simulink model "CLRFSPFCRealizedSimscape"  (R2024a)
settings: Solver=FixedStepAuto  StartTime=0.0  StopTime=0.1  FixedStep=1e-7  MaxStep=1e-6  RelTol=1e-3
undefined symbols (not defined in the file or in its folder): Rc1, Rc2, Rc3, Rclp, Rin1, Rin2, Rin3, Rout, Rst1, Rst2, Vc, vr
libraries: fl_lib x44, nesl_utility x9, ee_lib x5
settings Model: Creator=FactCore  LastModifiedBy=FactCore
settings SolverCC: ZeroCrossAlgorithm=Adaptive

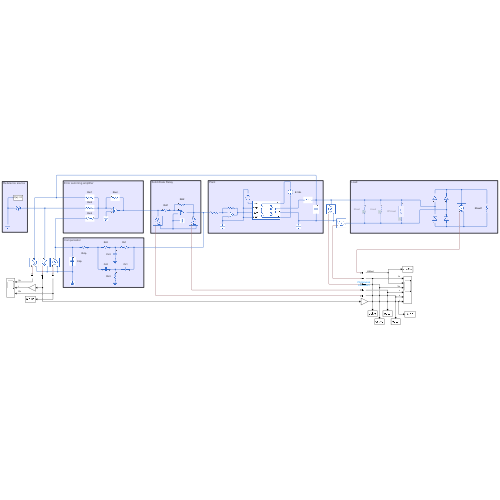
[thumbnail: Simulink's stored preview of the top-level diagram]
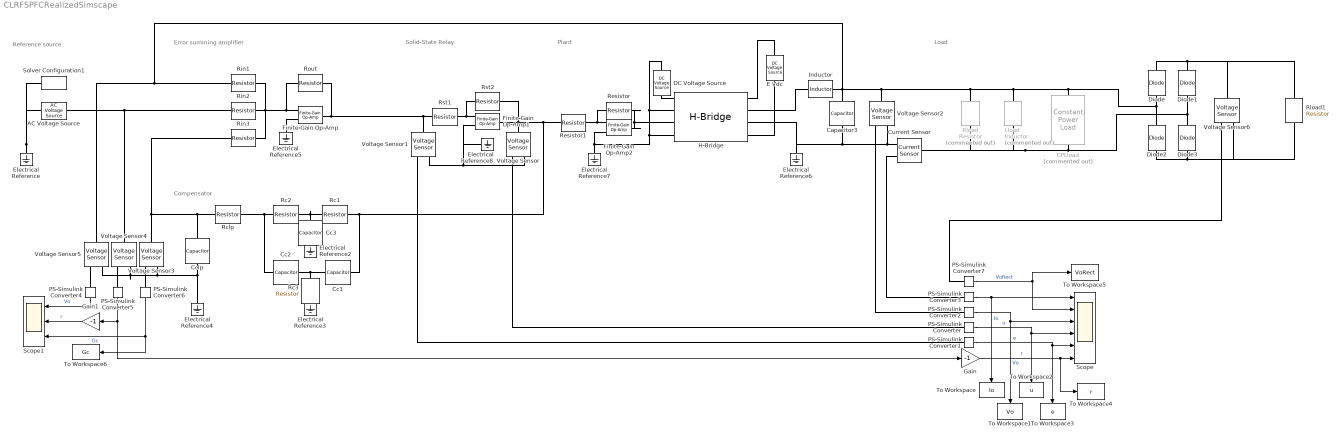
== system CLRFSPFCRealizedSimscape ==
  note: Reference source
  note: Error summing amplifier
  note: Compensator
  note: Load
  note: Plant
  note: Solid-State Relay
  AC Voltage Source : fl_lib/Electrical/Electrical Sources/AC Voltage Source  amp=vr*sqrt(2) V  shift=0 deg  frequency=fg Hz
  CPLload : ee_lib/Passive/Constant Power Load  Commented=on  load_type=ee.enum.dc_ac.ac  consumed_power=100 W  min_supply_voltage=20 V  G_reverse=1e-6 S  deltaV=1e-3 V  active_power=400 W  reactive_power=0 A*V  f0=fg Hz  Vrms_min=vr*0.85 V  tau=0.01 s  Vrms_ini=vr V  Vang_ini=0 deg  enable_fault=simscape.enum.onoff.off  fault_action=simscape.enum.assert.action.none  t_fault=1 s  open_conductance=1e-4 S
      settings: InternalSimscapePortConfiguration="{\"Bottom\":[],\"Left\":[{\"id\":\"p\",\"label\":\"+\",\"type\":\"foundation.electrical.electrical\"}],\"Right\":[{\"id\":\"n\",\"label\":\"-\",\"type\":\"foundation.electrical.electrical\"}],\"Top\":[]}"
  Capacitor3 : fl_lib/Electrical/Electrical Elements/Capacitor  c=Cf F  r=1e-6 Ohm  g=0 1/Ohm  i_specify=off  i_priority=None  i=0 A  i_nominal_specify=off  i_nominal_value=1  i_nominal_unit=A  v_specify=off  v_priority=None  v=0 V  v_nominal_specify=off  v_nominal_value=1  v_nominal_unit=V  vc_specify=off  vc_priority=High  vc=0 V  vc_nominal_specify=off  vc_nominal_value=1  vc_nominal_unit=V
  Cc1 : fl_lib/Electrical/Electrical Elements/Capacitor  c=Cc1 F  r=1e-6 Ohm  g=0 1/Ohm  i_specify=off  i_priority=None  i=0 A  i_nominal_specify=off  i_nominal_value=1  i_nominal_unit=A  v_specify=off  v_priority=None  v=0 V  v_nominal_specify=off  v_nominal_value=1  v_nominal_unit=V  vc_specify=off  vc_priority=High  vc=0 V  vc_nominal_specify=off  vc_nominal_value=1  vc_nominal_unit=V
  Cc2 : fl_lib/Electrical/Electrical Elements/Capacitor  c=Cc2 F  r=1e-6 Ohm  g=0 1/Ohm  i_specify=off  i_priority=None  i=0 A  i_nominal_specify=off  i_nominal_value=1  i_nominal_unit=A  v_specify=off  v_priority=None  v=0 V  v_nominal_specify=off  v_nominal_value=1  v_nominal_unit=V  vc_specify=off  vc_priority=High  vc=0 V  vc_nominal_specify=off  vc_nominal_value=1  vc_nominal_unit=V
  Cc3 : fl_lib/Electrical/Electrical Elements/Capacitor  c=Cc3 F  r=1e-6 Ohm  g=0 1/Ohm  i_specify=off  i_priority=None  i=0 A  i_nominal_specify=off  i_nominal_value=1  i_nominal_unit=A  v_specify=off  v_priority=None  v=0 V  v_nominal_specify=off  v_nominal_value=1  v_nominal_unit=V  vc_specify=off  vc_priority=High  vc=0 V  vc_nominal_specify=off  vc_nominal_value=1  vc_nominal_unit=V
  Cclp : fl_lib/Electrical/Electrical Elements/Capacitor  c=Cclp F  r=1e-6 Ohm  g=0 1/Ohm  i_specify=off  i_priority=None  i=0 A  i_nominal_specify=off  i_nominal_value=1  i_nominal_unit=A  v_specify=off  v_priority=None  v=0 V  v_nominal_specify=off  v_nominal_value=1  v_nominal_unit=V  vc_specify=off  vc_priority=High  vc=0 V  vc_nominal_specify=off  vc_nominal_value=1  vc_nominal_unit=V
  Current Sensor : fl_lib/Electrical/Electrical Sensors/Current Sensor
  DC Voltage Source : fl_lib/Electrical/Electrical Sources/DC Voltage Source  v0=5 V
  Diode{,1..3} (4 alike) : fl_lib/Electrical/Electrical Elements/Diode  Vf=0.6 V  Ron=0.3 Ohm  Goff=1e-8 1/Ohm  i_specify=off  i_priority=None  i=0 A  i_nominal_specify=off  i_nominal_value=1  i_nominal_unit=A  v_specify=off  v_priority=None  v=0 V  v_nominal_specify=off  v_nominal_value=1  v_nominal_unit=V
  E Vdc : fl_lib/Electrical/Electrical Sources/DC Voltage Source  v0=E V
  Electrical Reference{,2..8} (8 alike) : fl_lib/Electrical/Electrical Elements/Electrical Reference
  Finite-Gain Op-Amp : ee_lib/Integrated Circuits/Finite-Gain Op-Amp  A=1e4  Rin=1e6 Ohm  Rout=0.3 Ohm  Vmin=-Vc V  Vmax=Vc V  noise_mode=ee.enum.mode.disabled  v_noise=30e-9 V/Hz^(1/2)  noise_prm=ee.enum.ic.noiseParameterization.same  i_noise=0.5e-12 A/Hz^(1/2)  ip_noise=0.5e-12 A/Hz^(1/2)  in_noise=0.5e-12 A/Hz^(1/2)  sample_time=1e-3 s  repeatability=ee.enum.ic.repeatability.notRepeatable  auto_seed_v=545404223  auto_seed_ip=3922919431  auto_seed_in=2715962282  user_seed_v=0  user_seed_ip=0  user_seed_in=0
      settings: InternalSimscapePortConfiguration="{\"Bottom\":[],\"Left\":[{\"id\":\"p\",\"label\":\"+\",\"type\":\"foundation.electrical.electrical\"},{\"id\":\"n\",\"label\":\"-\",\"type\":\"foundation.electrical.electrical\"}],\"Right\":[{\"id\":\"out\",\"label\":\"\",\"type\":\"foundation.electrical.electrical\"}],\"Top\":[]}"
  Finite-Gain Op-Amp1 : ee_lib/Integrated Circuits/Finite-Gain Op-Amp  A=1e9  Rin=1e6 Ohm  Rout=0.3 Ohm  Vmin=-Vc V  Vmax=Vc V  noise_mode=ee.enum.mode.disabled  v_noise=30e-9 V/Hz^(1/2)  noise_prm=ee.enum.ic.noiseParameterization.same  i_noise=0.5e-12 A/Hz^(1/2)  ip_noise=0.5e-12 A/Hz^(1/2)  in_noise=0.5e-12 A/Hz^(1/2)  sample_time=1e-3 s  repeatability=ee.enum.ic.repeatability.notRepeatable  auto_seed_v=3437178441  auto_seed_ip=609397185  auto_seed_in=1811450916  user_seed_v=0  user_seed_ip=0  user_seed_in=0
      settings: InternalSimscapePortConfiguration="{\"Bottom\":[],\"Left\":[{\"id\":\"p\",\"label\":\"+\",\"type\":\"foundation.electrical.electrical\"},{\"id\":\"n\",\"label\":\"-\",\"type\":\"foundation.electrical.electrical\"}],\"Right\":[{\"id\":\"out\",\"label\":\"\",\"type\":\"foundation.electrical.electrical\"}],\"Top\":[]}"
  Finite-Gain Op-Amp2 : ee_lib/Integrated Circuits/Finite-Gain Op-Amp  A=1e4  Rin=1e6 Ohm  Rout=0.3 Ohm  Vmin=-Vc V  Vmax=Vc V  noise_mode=ee.enum.mode.disabled  v_noise=30e-9 V/Hz^(1/2)  noise_prm=ee.enum.ic.noiseParameterization.same  i_noise=0.5e-12 A/Hz^(1/2)  ip_noise=0.5e-12 A/Hz^(1/2)  in_noise=0.5e-12 A/Hz^(1/2)  sample_time=1e-3 s  repeatability=ee.enum.ic.repeatability.notRepeatable  auto_seed_v=2348838240  auto_seed_ip=4112460543  auto_seed_in=4144164703  user_seed_v=0  user_seed_ip=0  user_seed_in=0
      settings: InternalSimscapePortConfiguration="{\"Bottom\":[],\"Left\":[{\"id\":\"p\",\"label\":\"+\",\"type\":\"foundation.electrical.electrical\"},{\"id\":\"n\",\"label\":\"-\",\"type\":\"foundation.electrical.electrical\"}],\"Right\":[{\"id\":\"out\",\"label\":\"\",\"type\":\"foundation.electrical.electrical\"}],\"Top\":[]}"
  Gain : Gain  Gain=-1
  Gain1 : Gain  Gain=-1
  H-Bridge : ee_lib/Semiconductors & Converters/Converters/H-Bridge  supply_ports=ee.enum.supply_ports.showsupply  pwm_or_av=ee.enum.pwm_or_av.pwm  regenerative_braking_mode=ee.enum.converters.regenerative_braking_mode.depends_on_rev  discontinuous=ee.enum.current_profile.continuous  freewheeling_mode=ee.enum.converters.freewheeling_mode.one_switch_one_diode  Rload=10 Ohm  Lload=1e-5 H  F=10 kHz  Venable=2.5 V  Vmax=5.0 V  Vreverse=0.1 V  Vbrake=2.5 V  Vm=12 V  Ron=0.1 Ohm  Don=0.05 Ohm  Goff=1e-6 S  Tmeas=298.15 K  Ron2=0.1 Ohm  Don2=0.05 Ohm  Tmeas2=398.15 K  thermal_mass=100 J/K  initial_temperature=298.15 K
      settings: InternalSimscapePortConfiguration="{\"Bottom\":[],\"Left\":[{\"id\":\"ENA\",\"label\":\"PWM\",\"type\":\"foundation.electrical.electrical\"},{\"id\":\"REF\",\"label\":\"REF\",\"type\":\"foundation.electrical.electrical\"},{\"id\":\"REV\",\"label\":\"REV\",\"type\":\"foundation.electrical.electrical\"},{\"id\":\"BRK\",\"label\":\"BRK\",\"type\":\"foundation.electrical.electrical\"}],\"Right\":[{\"id\":\"p1\",\"label\":\"V+\",\"type\":\"foundation.electrical.electrical\"},{\"id\":\"p2\",\"label\":\"+\",\"type\":\"foundation.electrical.electrical\"},{\"id\":\"n2\",\"label\":\"-\",\"type\":\"foundation.electrical.electrical\"},{\"id\":\"n1\",\"label\":\"V-\",\"type\":\"foundation.electrical.electrical\"}],\"Top\":[]}"
  Inductor : fl_lib/Electrical/Electrical Elements/Inductor  l=Lf H  r=Rf Ohm  g=1e-9 1/Ohm  i_specify=off  i_priority=None  i=0 A  i_nominal_specify=off  i_nominal_value=1  i_nominal_unit=A  v_specify=off  v_priority=None  v=0 V  v_nominal_specify=off  v_nominal_value=1  v_nominal_unit=V  i_L_specify=off  i_L_priority=High  i_L=0 A  i_L_nominal_specify=off  i_L_nominal_value=1  i_L_nominal_unit=A
  Lload : fl_lib/Electrical/Electrical Elements/Inductor  Commented=on  l=400e-3 H  r=1 Ohm  g=1e-9 1/Ohm  i_specify=off  i_priority=None  i=0 A  i_nominal_specify=off  i_nominal_value=1  i_nominal_unit=A  v_specify=off  v_priority=None  v=0 V  v_nominal_specify=off  v_nominal_value=1  v_nominal_unit=V  i_L_specify=off  i_L_priority=High  i_L=0 A  i_L_nominal_specify=off  i_L_nominal_value=1  i_L_nominal_unit=A
  PS-Simulink Converter{,1..7} (8 alike) : nesl_utility/PS-Simulink Converter  PhysicalDomain=network_engine_domain  SubClassName=ps_output  LeftPortType=input  RightPortType=output  PseudoPeriodic=off  Frequencies=[]  VectorFormat=inherit  Unit=inherit  AffineConversion=off
  Rc1 : fl_lib/Electrical/Electrical Elements/Resistor  R=Rc1 Ohm  i_specify=off  i_priority=None  i=0 A  i_nominal_specify=off  i_nominal_value=1  i_nominal_unit=A  v_specify=off  v_priority=None  v=0 V  v_nominal_specify=off  v_nominal_value=1  v_nominal_unit=V
  Rc2 : fl_lib/Electrical/Electrical Elements/Resistor  R=Rc2 Ohm  i_specify=off  i_priority=None  i=0 A  i_nominal_specify=off  i_nominal_value=1  i_nominal_unit=A  v_specify=off  v_priority=None  v=0 V  v_nominal_specify=off  v_nominal_value=1  v_nominal_unit=V
  Rc3 : fl_lib/Electrical/Electrical Elements/Resistor  R=Rc3 Ohm  i_specify=off  i_priority=None  i=0 A  i_nominal_specify=off  i_nominal_value=1  i_nominal_unit=A  v_specify=off  v_priority=None  v=0 V  v_nominal_specify=off  v_nominal_value=1  v_nominal_unit=V
  Rclp : fl_lib/Electrical/Electrical Elements/Resistor  R=Rclp Ohm  i_specify=off  i_priority=None  i=0 A  i_nominal_specify=off  i_nominal_value=1  i_nominal_unit=A  v_specify=off  v_priority=None  v=0 V  v_nominal_specify=off  v_nominal_value=1  v_nominal_unit=V
  Resistor : fl_lib/Electrical/Electrical Elements/Resistor  R=10e3 Ohm  i_specify=off  i_priority=None  i=0 A  i_nominal_specify=off  i_nominal_value=1  i_nominal_unit=A  v_specify=off  v_priority=None  v=0 V  v_nominal_specify=off  v_nominal_value=1  v_nominal_unit=V
  Resistor1 : fl_lib/Electrical/Electrical Elements/Resistor  R=10e3 Ohm  i_specify=off  i_priority=None  i=0 A  i_nominal_specify=off  i_nominal_value=1  i_nominal_unit=A  v_specify=off  v_priority=None  v=0 V  v_nominal_specify=off  v_nominal_value=1  v_nominal_unit=V
  Rin1 : fl_lib/Electrical/Electrical Elements/Resistor  R=Rin1 Ohm  i_specify=off  i_priority=None  i=0 A  i_nominal_specify=off  i_nominal_value=1  i_nominal_unit=A  v_specify=off  v_priority=None  v=0 V  v_nominal_specify=off  v_nominal_value=1  v_nominal_unit=V
  Rin2 : fl_lib/Electrical/Electrical Elements/Resistor  R=Rin2 Ohm  i_specify=off  i_priority=None  i=0 A  i_nominal_specify=off  i_nominal_value=1  i_nominal_unit=A  v_specify=off  v_priority=None  v=0 V  v_nominal_specify=off  v_nominal_value=1  v_nominal_unit=V
  Rin3 : fl_lib/Electrical/Electrical Elements/Resistor  R=Rin3 Ohm  i_specify=off  i_priority=None  i=0 A  i_nominal_specify=off  i_nominal_value=1  i_nominal_unit=A  v_specify=off  v_priority=None  v=0 V  v_nominal_specify=off  v_nominal_value=1  v_nominal_unit=V
  Rload : fl_lib/Electrical/Electrical Elements/Resistor  Commented=on  R=150 Ohm  i_specify=off  i_priority=None  i=0 A  i_nominal_specify=off  i_nominal_value=1  i_nominal_unit=A  v_specify=off  v_priority=None  v=0 V  v_nominal_specify=off  v_nominal_value=1  v_nominal_unit=V
  Rload1 : fl_lib/Electrical/Electrical Elements/Resistor  R=150 Ohm  i_specify=off  i_priority=None  i=0 A  i_nominal_specify=off  i_nominal_value=1  i_nominal_unit=A  v_specify=off  v_priority=None  v=0 V  v_nominal_specify=off  v_nominal_value=1  v_nominal_unit=V
  Rout : fl_lib/Electrical/Electrical Elements/Resistor  R=Rout Ohm  i_specify=off  i_priority=None  i=0 A  i_nominal_specify=off  i_nominal_value=1  i_nominal_unit=A  v_specify=off  v_priority=None  v=0 V  v_nominal_specify=off  v_nominal_value=1  v_nominal_unit=V
  Rst1 : fl_lib/Electrical/Electrical Elements/Resistor  R=Rst1 Ohm  i_specify=off  i_priority=None  i=0 A  i_nominal_specify=off  i_nominal_value=1  i_nominal_unit=A  v_specify=off  v_priority=None  v=0 V  v_nominal_specify=off  v_nominal_value=1  v_nominal_unit=V
  Rst2 : fl_lib/Electrical/Electrical Elements/Resistor  R=Rst2 Ohm  i_specify=off  i_priority=None  i=0 A  i_nominal_specify=off  i_nominal_value=1  i_nominal_unit=A  v_specify=off  v_priority=None  v=0 V  v_nominal_specify=off  v_nominal_value=1  v_nominal_unit=V
  Scope : Scope  NumInputPorts=6
  Scope1 : Scope  NumInputPorts=3
  Solver Configuration1 : nesl_utility/Solver Configuration  PhysicalDomain=network_engine_domain  SubClassName=solver  LeftPortType=input  RightPortType=generic  Tones=[]  Harmonics=[]  SimulateNoise=off  Profile=off  UseLocalSampling=off  EnableSwitchedLinearOptims=on  FrequencyDomain=off  UseCCode=off  RelTol=0.001  AbsTol=0.001  MinStep=1e-09  ToWorkspace=off  RevertToSquareIcSolve=off  NumHomotopyIterations=100  PhasorMode=off  PhasorModeNumHarmonics=1  ConsistencySolver=NEWTON_XTOL_AFTER_FTOL  IndexReductionMethod=DerivativeReplacement  DoDC=off  ResidualTolerance=1e-09  ConsistencyTolSource=GLOBAL  ConsistencyAbsTol=0.001  ConsistencyRelTol=0.001  ConsistencyTolFactor=0.001  UseLocalSolver=off  LocalSolverChoice=NE_BACKWARD_EULER_ADVANCER  ResolveIndetEquations=on  FunctionEvalNumThread=1  LocalSolverSampleTime=0.001  DoFixedCost=off  MaxNonlinIter=3  MaxModeIter=2  ComputeImpulses=off  ImpulseIterations=2  LinearAlgebra=auto  LinearAlgebraNumThread=0  EquationFormulation=NE_TIME_EF  DelaysMemoryBudget=4096  AutomaticFiltering=on  FilteringTimeConstant=0.001  PartitionStorageMethod=AS_NEEDED  PartitionMemoryBudget=1024  PartitionMethod=ROBUST  MultibodyUseLocalSolver=off  MultibodyLocalSolverChoice=ODE1  MultibodyLocalSolverSampleTime=0.001
  To Workspace : ToWorkspace  VariableName=Io  SampleTime=-1
  To Workspace1 : ToWorkspace  VariableName=Vo  SampleTime=-1
  To Workspace2 : ToWorkspace  VariableName=u  SampleTime=-1
  To Workspace3 : ToWorkspace  VariableName=e  SampleTime=-1
  To Workspace4 : ToWorkspace  VariableName=r  SampleTime=-1
  To Workspace5 : ToWorkspace  VariableName=VoRect  SampleTime=-1
  To Workspace6 : ToWorkspace  VariableName=Gc  SampleTime=-1
  Voltage Sensor{,1..6} (7 alike) : fl_lib/Electrical/Electrical Sensors/Voltage Sensor
  wires:
  PS-Simulink Converter/1 -> To Workspace2/1, Scope/4  "u"
  PS-Simulink Converter1/1 -> To Workspace3/1, Scope/5  "e"
  PS-Simulink Converter2/1 -> Scope/3, To Workspace1/1  "Vo"
  PS-Simulink Converter3/1 -> Scope/1, To Workspace/1  "Io"
  PS-Simulink Converter4/1 -> Scope1/1  "Vo"
  PS-Simulink Converter6/1 -> Scope1/3, To Workspace6/1  "Gc"
  PS-Simulink Converter5/1 -> Gain/1, Gain1/1
  Gain/1 -> To Workspace4/1, Scope/6  "r"
  Gain1/1 -> Scope1/2  "r"
  PS-Simulink Converter7/1 -> To Workspace5/1, Scope/2  "VoRect"
  connections:
  Rst1/RConn1 -- Finite-Gain Op-Amp1/LConn1 -- Rst2/LConn1
  Voltage Sensor/RConn1 -- PS-Simulink Converter/LConn1
  PS-Simulink Converter1/LConn1 -- Voltage Sensor1/RConn1
  Electrical Reference/LConn1 -- Solver Configuration1/RConn1 -- AC Voltage Source/RConn1
  H-Bridge/LConn1 -- DC Voltage Source/LConn1
  Electrical Reference2/LConn1 -- Cc3/RConn1
  Electrical Reference3/LConn1 -- Rc3/RConn1
  E Vdc/LConn1 -- H-Bridge/RConn1
  H-Bridge/RConn4 -- E Vdc/RConn1
  Rc2/LConn1 -- Cc3/LConn1 -- Rc1/RConn1
  Cc1/RConn1 -- Cc2/LConn1 -- Rc3/LConn1
  Cc2/RConn1 -- Rclp/LConn1 -- Rc2/RConn1
  Cclp/LConn1 -- Rclp/RConn1 -- Rin3/LConn1 -- Voltage Sensor3/LConn1
  Voltage Sensor4/RConn2 -- Voltage Sensor5/RConn2 -- Voltage Sensor3/RConn2 -- Cclp/RConn1 -- Electrical Reference4/LConn1
  Voltage Sensor/RConn2 -- Voltage Sensor1/RConn2 -- Electrical Reference8/LConn1 -- Finite-Gain Op-Amp1/LConn2
  Rin2/RConn1 -- Rin3/RConn1 -- Rin1/RConn1 -- Rout/LConn1 -- Finite-Gain Op-Amp/LConn2
  PS-Simulink Converter2/LConn1 -- Voltage Sensor2/RConn1
  Current Sensor/RConn1 -- PS-Simulink Converter3/LConn1
  PS-Simulink Converter4/LConn1 -- Voltage Sensor5/RConn1
  PS-Simulink Converter5/LConn1 -- Voltage Sensor4/RConn1
  Voltage Sensor3/RConn1 -- PS-Simulink Converter6/LConn1
  Diode1/LConn1 -- Current Sensor/LConn1 -- Rload/RConn1 -- Lload/RConn1 -- CPLload/RConn1 -- Diode3/RConn1
  Finite-Gain Op-Amp/LConn1 -- Electrical Reference5/LConn1
  Finite-Gain Op-Amp/RConn1 -- Rout/RConn1 -- Rst1/LConn1 -- Voltage Sensor1/LConn1
  Rc1/LConn1 -- Finite-Gain Op-Amp1/RConn1 -- Rst2/RConn1 -- Voltage Sensor/LConn1 -- Resistor1/LConn1 -- Cc1/LConn1
  H-Bridge/RConn2 -- Inductor/LConn1
  Voltage Sensor4/LConn1 -- AC Voltage Source/LConn1 -- Rin2/LConn1
  Finite-Gain Op-Amp2/RConn1 -- H-Bridge/LConn3 -- Resistor/RConn1
  Finite-Gain Op-Amp2/LConn2 -- Resistor/LConn1 -- Resistor1/RConn1
  H-Bridge/LConn2 -- Finite-Gain Op-Amp2/LConn1 -- Electrical Reference7/LConn1 -- H-Bridge/LConn4 -- DC Voltage Source/RConn1
  Current Sensor/RConn2 -- Voltage Sensor2/RConn2 -- Capacitor3/RConn1 -- H-Bridge/RConn3 -- Electrical Reference6/LConn1
  Diode/RConn1 -- Voltage Sensor6/LConn1 -- Rload1/LConn1 -- Diode1/RConn1
  Diode2/LConn1 -- Voltage Sensor6/RConn2 -- Rload1/RConn1 -- Diode3/LConn1
  Inductor/RConn1 -- Lload/LConn1 -- CPLload/LConn1 -- Diode2/RConn1 -- Diode/LConn1 -- Rload/LConn1 -- Voltage Sensor2/LConn1 -- Capacitor3/LConn1 -- Rin1/LConn1 -- Voltage Sensor5/LConn1
  PS-Simulink Converter7/LConn1 -- Voltage Sensor6/RConn1
